simulink model "MyFirstModel"  (R2021a)
settings: Solver=VariableStepAuto  StartTime=0.0  StopTime=2  MaxStep=1e-3  RelTol=1e-3
libraries: simulink x1
settings Model: Creator=reemb  LastModifiedBy=reemb

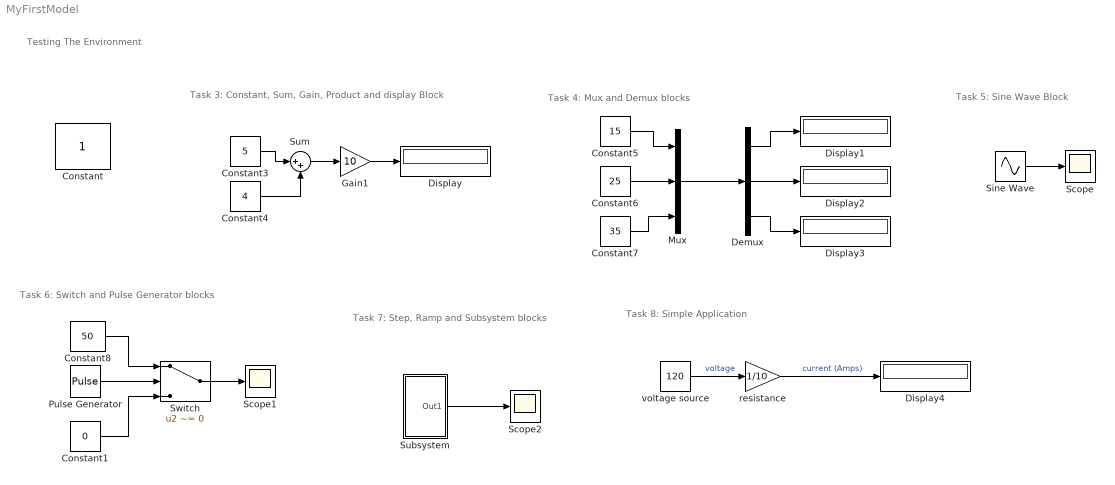
== system MyFirstModel ==
  note: Testing The Environment
  note: Task 3: Constant, Sum, Gain, Product and display Block
  note: Task 8: Simple Application
  note: Task 7: Step, Ramp and Subsystem blocks
  note: Task 4: Mux and Demux blocks
  note: Task 5: Sine Wave Block
  note: Task 6: Switch and Pulse Generator blocks
  Constant : Constant
  Constant1 : Constant  Value=0
  Constant3 : Constant  Value=5
  Constant4 : Constant  Value=4
  Constant5 : Constant  Value=15
  Constant6 : Constant  Value=25
  Constant7 : Constant  Value=35
  Constant8 : Constant  Value=50
  Demux : Demux  Outputs=3
  Display{,1..4} (5 alike) : Display
  Gain1 : Gain  Gain=10
  Mux : Mux  Inputs=3
  Pulse Generator : DiscretePulseGenerator  PulseType=Time based  Period=10  PulseWidth=5
  Scope : Scope
  Scope1 : Scope
  Scope2 : Scope
  Sine Wave : Sin  Amplitude=10  Frequency=2*pi *5  SampleTime=0
  Subsystem : Subsystem
  Sum : Sum  Inputs=|++
  Switch : Switch  Criteria=u2 ~= 0
  resistance : Gain  Gain=1/10
  voltage source : Constant  Value=120
  wires:
  Sine Wave/1 -> Scope/1
  Constant5/1 -> Mux/1
  Demux/3 -> Display3/1
  Demux/2 -> Display2/1
  Mux/1 -> Demux/1
  Constant7/1 -> Mux/3
  Demux/1 -> Display1/1
  Constant6/1 -> Mux/2
  Constant3/1 -> Sum/1
  Constant4/1 -> Sum/2
  Sum/1 -> Gain1/1
  Gain1/1 -> Display/1
  Pulse Generator/1 -> Switch/2
  Constant8/1 -> Switch/1
  Constant1/1 -> Switch/3
  Switch/1 -> Scope1/1
  Subsystem/1(Out1) -> Scope2/1
  voltage source/1 -> resistance/1  "voltage"
  resistance/1 -> Display4/1  "current (Amps)"

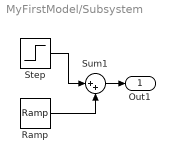
== system MyFirstModel/Subsystem ==
  Ramp : simulink/Sources/Ramp  slope=2  start=0  InitialOutput=0
  Step : Step  After=10  SampleTime=0
  Sum1 : Sum  Inputs=|++
  Out1 : Outport
  wires:
  Ramp/1 -> Sum1/2
  Step/1 -> Sum1/1
  Sum1/1 -> Out1/1
